simulink model "FINAL_AUTO_PHASE_2_V4"  (R2020b)
settings: Solver=ode23t  StartTime=0.0  StopTime=180.1  FixedStep=0.05  RelTol=1e-3  EnableMultiTasking=on
model workspace (MAT data in the model file):
  DROP_VACCINE_TIME = 0.25
  GRID_SIDE = 0.457142857143
  HALF_TICKS_TO_DIST = 0.00174532925
  LATCHER_OFFSET = 0.3934603175
  LATCH_CELL_TIME = 0.5
  LOWER_PLATFORM_TIME = 0.5
  NUM_SURVEY_GRIDS = 7
  SPACE_SIDE = 0.152380952381
  SURVEY_GRIDS_CELLS : Simulink.Signal (value not decoded)
  SURVEY_GRIDS_COORDS = [5 5 5 4 5 5 6 6 5 4 3 2 ... (14 elements, 7x2)]
  SURVEY_TURN_ANGLE = 22.7856177106
  WAIT_CONFIRM_CELL_TIME = 0.08
  mapForSim : object (value not decoded)
  occGrid : robotics.BinaryOccupancyGrid (value not decoded)
  oldDetectedCellType : Simulink.Signal (value not decoded)
  unsavedUninfectedCells : Simulink.Signal (value not decoded)
undefined symbols (not defined in the file): cellLevel, cellPose, cellTypeArray, FloorSurface, isoPoses, platformPoses, PlowSurface, Ref, RobotSurface, WallSurface, X, Y, Z
libraries: sm_lib x286, nesl_utility x157, simulink x72, pid_lib x3
(part 15 of 15)

== stateflow chart FINAL_AUTO_PHASE_2_V4/stateflow MAIN_PROGRAM ==
  state MAIN_PROGRAM
    state PHASE_1
      state DROP_VAC_1
      state DROP_VAC_2
      state CLEAR_PLATFORM_1
      state DROP_VAC_3
      state CLEAR_PLATFORM_2
      (default) -> DROP_VAC_1
      DROP_VAC_1 -> DROP_VAC_2 : [hasDroppedVacAt(0.9904761905, 0.8380952381)]
      DROP_VAC_2 -> CLEAR_PLATFORM_1 : [hasDroppedVacAt(1.0404761905, 2.361904762)]
      CLEAR_PLATFORM_1 -> DROP_VAC_3 : [hasClearedPlatformAt(5, 5)]
      DROP_VAC_3 -> CLEAR_PLATFORM_2 : [hasDroppedVacAt(2.361904762, 1.752380952)]
    state PAHSE_2
      state EVACUATE_UNINFECTED_CELLS
      state AUTONOMOUS_COMPLETED
        entry:
        leftMotor = 0
        rightMotor = 0
      (default) -> EVACUATE_UNINFECTED_CELLS
      EVACUATE_UNINFECTED_CELLS -> AUTONOMOUS_COMPLETED : [hasSavedAllUninfected()]
    state deliveredVac = hasDroppedVacAt(xCoord, yCoord) [function]
    state platformCleared = hasClearedPlatformAt(gridX,gridY) [function]
    state allUninfectedSaved = hasSavedAllUninfected [function]
    (default) -> PHASE_1
    CLEAR_PLATFORM_2 -> PAHSE_2 : [hasClearedPlatformAt(6, 0)]
  (default) -> MAIN_PROGRAM
  data: xCoord function_input double size=1; yCoord function_input double size=1; deliveredVac function_output; gridX function_input double size=1; gridY function_input double size=1; platformCleared function_output; allUninfectedSaved function_output; rightMotor data_store_memory; leftMotor data_store_memory

== matlab function FINAL_AUTO_PHASE_2_V4/BEST Robotics 2020 Game (Double-Click)/Vaccines/Vaccine1/MATLAB Function1 ==
  settings: updateMethod=DISCRETE
  data: drop input; level input; objPoseX output; robotPoseX input; robotPoseY input; objPoseY output; vaccine output
function [objPoseX, objPoseY, vaccine] = latchObject(drop, level, robotPoseX, robotPoseY)
persistent stateX stateY stateZ prevDrop dropped
if isempty(stateX)
    stateX=robotPoseX+0.14;
    stateY=robotPoseY;
    stateZ=0.15;
    prevDrop=0;
    dropped=0;
end

if drop && prevDrop && ~dropped
    stateX=robotPoseX;
    stateY=robotPoseY;
    stateZ=level*0.4;
    objPoseX=robotPoseX;
    objPoseY=robotPoseY;
    dropped=1;
elseif dropped
    objPoseX=stateX;
    objPoseY=stateY;

else
    objPoseX=robotPoseX-0.11;
    objPoseY=robotPoseY-0.11;
end
prevDrop=drop;
vaccine=stateZ;

== matlab function FINAL_AUTO_PHASE_2_V4/function getFullRobotAngle ==
  data: robotAngle input; fullRobotAngle input; fullRobotAngle output; leftTicks input; rightTicks input; prevLTicks input; prevRTicks input
function fullRobotAngle = getFullRobotAngle(robotAngle, fullRobotAngle, ...
    leftTicks, rightTicks, prevLTicks, prevRTicks)

% just choose one of the encoder tick differences, since
    % the motors always have the same speed
% the weird decimal is the change in degrees per encoder tick
angleChange = abs(leftTicks - prevLTicks) * 0.7804878049;

% if the robot is turning clockwise
if leftTicks > prevLTicks && rightTicks < prevRTicks
    fullRobotAngle = fullRobotAngle - angleChange;
% if the robot is turning counter-clockwise
elseif rightTicks > prevRTicks && leftTicks < prevLTicks
    fullRobotAngle = fullRobotAngle + angleChange;
end

% normalize the angle to be 0 to 359 degrees
if fullRobotAngle >= 360
    fullRobotAngle = mod(fullRobotAngle, 360);
elseif fullRobotAngle < 0
    fullRobotAngle = fullRobotAngle + 360;
end

% last-minute (ngl kinda janky) angle correction 
if abs(fullRobotAngle - robotAngle) ... 
        < abs(fullRobotAngle - (360 - robotAngle))
    fullRobotAngle = robotAngle;
else
    fullRobotAngle = 360 - robotAngle;
end

== stateflow chart FINAL_AUTO_PHASE_2_V4/stateflow MAIN_PROGRAM/MAIN_PROGRAM.hasDroppedVacAt/Stateflow ==
  state DROP_VACCINE
    entry:
    leftMotor = 0
    rightMotor = 0
    dropVaccine()
  state MOVE_TO_VAC_SQUARE
    entry:
    vaccineDropped = false
  state COOL_VACCINE_DROP
    entry: vaccineDropped = true
  (default) -> MOVE_TO_VAC_SQUARE
  MOVE_TO_VAC_SQUARE -> DROP_VACCINE : [hasMovedToCoords(xCoord, yCoord, 0)]
  DROP_VACCINE -> COOL_VACCINE_DROP : [after(DROP_VACCINE_TIME, sec)]
  COOL_VACCINE_DROP -> MOVE_TO_VAC_SQUARE
  data: xCoord input; yCoord input; vaccineDropped output; leftMotor data_store_memory; rightMotor data_store_memory; DROP_VACCINE_TIME parameter

== matlab function FINAL_AUTO_PHASE_2_V4/function surveySweepHasFoundCell/function cellCriteriaFound/function cellCriteriaFound ==
  data: onlyUninfected input; cellFound output; detectedCellType data_store_memory
function cellFound = cellCriteriaFound(onlyUninfected)

global detectedCellType;

cellFound = false;
if ~isnan(detectedCellType)
   if onlyUninfected 
      cellFound = detectedCellType == 0; 
   else
       cellFound = true;
   end
end

== stateflow chart FINAL_AUTO_PHASE_2_V4/function hasTurnedToAngle/stateflow integrateSettleTime ==
  state ELAPSE_SETTLE_TIME
    during:
    settledTime = settledTime + 1
  state RESET_SETTLE_TIME
    entry:
    settledTime = 0
  (default) -> RESET_SETTLE_TIME
  RESET_SETTLE_TIME -> ELAPSE_SETTLE_TIME : [error <= TOLERANCE]
  ELAPSE_SETTLE_TIME -> RESET_SETTLE_TIME : [error > TOLERANCE]
  data: TOLERANCE input; error input; settledTime data_store_memory

== stateflow chart FINAL_AUTO_PHASE_2_V4/function hasMovedToCoords/stateflow hasMovedToCoords ==
  state CALCULATE_PATH
    entry:
    currentSurveyGridIndex = 0
    hasArrived = false
    changeX = xCoord - xPos
    changeY = yCoord - yPos
    targetAngle = normalizeAngle(...
    atand(changeY / changeX), changeX)
    wantedDist = getDist(changeX, changeY, useRobotPos)
    oldXCoord = xCoord
    oldYCoord = yCoord
  state TURN_TO_TARGET
  state DRIVE_TO_TARGET
  state HAS_ARRIVED
    entry:
    hasArrived = true
  (default) -> CALCULATE_PATH
  CALCULATE_PATH -> TURN_TO_TARGET
  TURN_TO_TARGET -> DRIVE_TO_TARGET : [hasTurnedToAngle(targetAngle)]
  DRIVE_TO_TARGET -> HAS_ARRIVED : [hasMovedDist(wantedDist)]
  HAS_ARRIVED -> CALCULATE_PATH : [xCoord ~= oldXCoord || yCoord ~= oldYCoord]
  data: angle function_output; angle function_input; xChange function_input; targetDist function_output double size=1; xChange function_input; yChange function_input; usingRobotPos function_input; LATCHER_OFFSET parameter size=1; xCoord input; yCoord input; targetAngle local; xPos data_store_memory; yPos data_store_memory; hasArrived output; oldYCoord local; oldXCoord local; changeY local; changeX local; useRobotPos input; wantedDist local; currentSurveyGridIndex data_store_memory
  function angle = normalizeAngle(angle, xChange):
    | function angle = normalizeAngle(angle, xChange)
    | 
    | if xChange < 0
    |     angle = angle + 180;
    | end
  function targetDist = getDist(xChange, yChange, usingRobotPos):
    | function targetDist = getDist(xChange, yChange, usingRobotPos)
    |  
    | targetDist = sqrt(xChange^2 + yChange^2);
    | 
    | if ~usingRobotPos
    |     % the weird decimal is the constant distance 
    |     % between the latcher xy and the robot xy
    |     targetDist = targetDist - LATCHER_OFFSET;
    | end

== stateflow chart FINAL_AUTO_PHASE_2_V4/function hasMovedDist/stateflow postSettleDist ==
  state SETTLE
  state RESET_DIST_AFTER_SETTLE
    entry:
    leftMotor = 0
    rightMotor = 0
    resetLeftEncoder = 1
    resetRightEncoder = 1
    straightDistTraveled = 0
    resetLeftEncoder = 0
    resetRightEncoder = 0
  (default) -> SETTLE
  RESET_DIST_AFTER_SETTLE -> SETTLE
  SETTLE -> RESET_DIST_AFTER_SETTLE : [distHasSettled]
  data: distHasSettled input; resetLeftEncoder data_store_memory; resetRightEncoder data_store_memory; straightDistTraveled data_store_memory; leftMotor data_store_memory; rightMotor data_store_memory

== matlab function FINAL_AUTO_PHASE_2_V4/function hasMovedDist/function getMoveDirSign ==
  data: u input double size=1; sign output double size=1
function sign = getMoveDirSign(u)

if u > 0
    sign = 1;
elseif u < 0
    sign = -1;
else
    sign = 0;
end

== stateflow chart FINAL_AUTO_PHASE_2_V4/function hasMovedDist/stateflow integrateSettleTime ==
  state ELAPSE_SETTLE_TIME
    during:
    settledTime = settledTime + 1
  state RESET_SETTLE_TIME
    entry:
    settledTime = 0
  (default) -> RESET_SETTLE_TIME
  RESET_SETTLE_TIME -> ELAPSE_SETTLE_TIME : [error <= TOLERANCE]
  ELAPSE_SETTLE_TIME -> RESET_SETTLE_TIME : [error > TOLERANCE]
  data: TOLERANCE input; error input; settledTime data_store_memory

== matlab function FINAL_AUTO_PHASE_2_V4/function updateCurrentSurveyGridIndex ==
  data: SURVEY_GRIDS_CELLS data_store_memory; detectedCellType data_store_memory; oldDetectedCellType data_store_memory; currentSurveyGridIndex data_store_memory; GRID_SIDE parameter; NUM_SURVEY_GRIDS parameter; SURVEY_GRIDS_COORDS parameter; latchCell data_store_memory
function updateCurrentSurveyGridIndex(GRID_SIDE, NUM_SURVEY_GRIDS, SURVEY_GRIDS_COORDS)

global latchCell;
global detectedCellType;
global currentSurveyGridIndex;

if ~latchCell && ~isnan(detectedCellType)
    % initialize the minimum-iterator for-loop with the distance to the first
    % survey grid-square
    closestGridSquare = 1;

    % use a reasonably formulaic value to give us a crazy value for
    % initializing the discovered minimum distance to a survey grid-sqaure
    minDist = GRID_SIDE;

    for iii = 1:NUM_SURVEY_GRIDS
        currentDist = getDistToGrid(SURVEY_GRIDS_COORDS(iii, 1), SURVEY_GRIDS_COORDS(iii, 2));
        if currentDist < minDist && currentDist < GRID_SIDE
            minDist = currentDist;
            closestGridSquare = iii;
        end
    end

    % use 0 as the null value in case the closest survey grid-square we're
    % occupying is too far, meaning at least one grid-square length away
    if minDist >= GRID_SIDE
        closestGridSquare = 0;
    end

    currentSurveyGridIndex = closestGridSquare;
end

== matlab function FINAL_AUTO_PHASE_2_V4/function getCoordChanges ==
  data: changeInDist input; fullRobotAngle input; newXPos output; newYPos output; xPos data_store_memory; yPos data_store_memory
function [newXPos, newYPos] = updateCoords(changeInDist, fullRobotAngle)
% assumes that the robot angle input is from 0 to 360 degrees

global xPos;
global yPos;

newXPos = xPos + (changeInDist * cosd(fullRobotAngle));
newYPos = yPos + (changeInDist * sind(fullRobotAngle));

== matlab function FINAL_AUTO_PHASE_2_V4/function hasSurveyedSides/function getSurveyAngles ==
  data: pivotSide input; firstSurveyAngle output; secondSurveyAngle output; SURVEY_TURN_ANGLE parameter; returnAngle output
function [firstSurveyAngle, secondSurveyAngle, returnAngle] ...
    = getSurveyAngles(pivotSide, SURVEY_TURN_ANGLE)

coder.extrinsic('MException')

switch pivotSide
    case 1
        firstSurveyAngle = 180.0 - SURVEY_TURN_ANGLE;
        secondSurveyAngle = 180.0 + SURVEY_TURN_ANGLE;
        returnAngle = 180;
    case 2
        firstSurveyAngle = 270.0 - SURVEY_TURN_ANGLE;
        secondSurveyAngle = 270.0 + SURVEY_TURN_ANGLE;
        returnAngle = 270;
    case 3
        firstSurveyAngle = SURVEY_TURN_ANGLE;
        secondSurveyAngle = 360.0 - SURVEY_TURN_ANGLE;
        returnAngle = 0;
    case 4
        firstSurveyAngle = 90.0 + SURVEY_TURN_ANGLE;
        secondSurveyAngle = 90.0 - SURVEY_TURN_ANGLE;
        returnAngle = 90;
    otherwise
        % use 0-angle values to visually show us there was something wrong
        % with finding the optimal rotated quadrant to approach the 
        % target grid-square from
        
        firstSurveyAngle = 0.0;
        secondSurveyAngle = 0.0;
        returnAngle = 0.0;
end

== matlab function FINAL_AUTO_PHASE_2_V4/function getDistChange ==
  data: leftTicks input; distChange output; rightTicks input; prevLTicks input; prevRTicks input; moveDir input; prevLTicks output; prevRTicks output; HALF_TICKS_TO_DIST parameter
function [distChange, prevLTicks, prevRTicks] ...
    = updateDistTraveled(leftTicks, rightTicks, ...
    prevLTicks, prevRTicks, moveDir, ...
    HALF_TICKS_TO_DIST)

% HALF_TICKS_TO_DIST = 0.5 * (2*pi*wheelRadius) / 180, wheelRadius = 0.1
distChange = ((leftTicks - prevLTicks) + (rightTicks - prevRTicks)) ...
    * (moveDir * HALF_TICKS_TO_DIST);

prevLTicks = leftTicks;
prevRTicks = rightTicks;

== matlab function FINAL_AUTO_PHASE_2_V4/function hasTurnedToAngle/function filterErrorAngle ==
  data: angleDiff input; optimalAngleDiff output
function optimalAngleDiff = filterErrorAngle(angleDiff)

if abs(angleDiff) > 180
    if angleDiff < 0
        optimalAngleDiff = angleDiff + 360;
    else
        optimalAngleDiff = angleDiff - 360;
    end
else
    optimalAngleDiff = angleDiff;
end

== matlab function FINAL_AUTO_PHASE_2_V4/function hasTurnedToAngle/function fixUserAngle ==
  data: targetAngle input; targetAngle output
function targetAngle = fixUserAngle(targetAngle)

% angle wrapper function to fix user input angle assumes
% an extreme input from -360 to 360

if targetAngle < 0 || targetAngle > 359
    % make sure to also include the truncated decimal part of the 
    % angle after applying modulus
    targetAngle = mod(targetAngle, 360) + (targetAngle - floor(targetAngle));
end

== matlab function FINAL_AUTO_PHASE_2_V4/function displayCellType ==
  data: cellType input; green output; orange output; red output
function [green, orange, red] = displayCellType(cellType)

green = 0;
orange = 0;
red = 0;

% Identify the detected cell type and lit up the corresponding lamp bit
if ~isnan(cellType)
    switch cellType
        case 0      % means uninfected
            orange = 1;
        case 1      % means vaccinated
            green = 1;
        case 2      % means infected
            red = 1;
    end   
end

== stateflow chart FINAL_AUTO_PHASE_2_V4/function hasSurveyedSides/stateflow hasSurveyedSides ==
  state FIRST_SURVEY_TURN
    entry:
    hasSurveyedSides = false
  state FIRST_CONFIRM_CELL
  state SECOND_SURVEY_TURN
  state SECOND_CONFIRM_CELL
  state RETURN_TO_PATH_ANGLE
  state SIDE_SURVEYING_DONE
    entry: hasSurveyedSides = true
  (default) -> FIRST_SURVEY_TURN
  SIDE_SURVEYING_DONE -> FIRST_SURVEY_TURN
  FIRST_SURVEY_TURN -> FIRST_CONFIRM_CELL : [hasTurnedToAngle(firstSurveyAngle)]
  FIRST_CONFIRM_CELL -> SECOND_SURVEY_TURN : [after(WAIT_CONFIRM_CELL_TIME, sec)]
  SECOND_SURVEY_TURN -> SECOND_CONFIRM_CELL : [hasTurnedToAngle(secondSurveyAngle)]
  SECOND_CONFIRM_CELL -> RETURN_TO_PATH_ANGLE : [after(WAIT_CONFIRM_CELL_TIME, sec)]
  RETURN_TO_PATH_ANGLE -> SIDE_SURVEYING_DONE : [hasTurnedToAngle(returnAngle)]
  data: firstSurveyAngle input; WAIT_CONFIRM_CELL_TIME parameter; secondSurveyAngle input; hasSurveyedSides output boolean size=1; returnAngle input

== matlab function FINAL_AUTO_PHASE_2_V4/Simulink Function/function getClosestValidGrid ==
  data: closestGridX output; closestGridY output; SURVEY_GRIDS_COORDS parameter; SURVEY_GRIDS_CELLS data_store_memory; closestGridIndex output; currentSurveyGridIndex data_store_memory; NUM_SURVEY_GRIDS parameter
function [closestGridX, closestGridY, closestGridIndex] ...
    = getClosestValidGrid(  SURVEY_GRIDS_COORDS, NUM_SURVEY_GRIDS)

global currentSurveyGridIndex;
global SURVEY_GRIDS_CELLS;

% initially invalid index should never cause an index error, because
% should always be a grid-square with at least one uninfected cell
% before we find all the available uninfected cells
closestGridIndex = 0;

% use the first grid-square (that we are not occupying) as the default
% initializer value for our linear min-dist-to-a-grid-square iteration
for iii = 1:NUM_SURVEY_GRIDS
    if iii ~= currentSurveyGridIndex
        closestGridIndex = iii;
        break
    end
end

closestGridX = SURVEY_GRIDS_COORDS(closestGridIndex, 1);
closestGridY = SURVEY_GRIDS_COORDS(closestGridIndex, 2);
minDist = getDistToGrid(closestGridX, closestGridY);
maxPossibleCells = max(SURVEY_GRIDS_CELLS);

for iii = 1:NUM_SURVEY_GRIDS
   currentGridX = SURVEY_GRIDS_COORDS(iii, 1);
   currentGridY = SURVEY_GRIDS_COORDS(iii, 2);
   distToIxSurveyGrid = getDistToGrid(currentGridX, currentGridY);
   if (iii ~= currentSurveyGridIndex && distToIxSurveyGrid < minDist) && ...
   SURVEY_GRIDS_CELLS(iii) == maxPossibleCells
      closestGridIndex = iii;
      minDist = distToIxSurveyGrid;
      closestGridX = currentGridX;
      closestGridY = currentGridY;
   end
end
